simulink model "ipi_model_comparison_template"  (R2020a)
settings: Solver=ode4  StartTime=0.0  StopTime=10.0  FixedStep=1E-3  RelTol=1e-3
values from neighbouring files (symbols this model uses):
  g = 9.81    [RMIC_traj_optim_config_start.m]
  l1 = 1    [RMIC_traj_optim_config_start.m]
  lc1 = l1/2    (= 0.5)    [RMIC_traj_optim_config_start.m]
  lc2 = l2/2    (= 0.5)    [RMIC_traj_optim_config_start.m]
  m1 = 10    [RMIC_traj_optim_config_start.m]
  m2 = 10    [RMIC_traj_optim_config_start.m]
undefined symbols (not defined in the file or in its folder): beta_b, I1zz, I2zz, X
settings Model: Creator=fernando  LastModifiedBy=User
settings SFSimCC: CustomCodeUndefinedFunction=UseInterfaceOnly

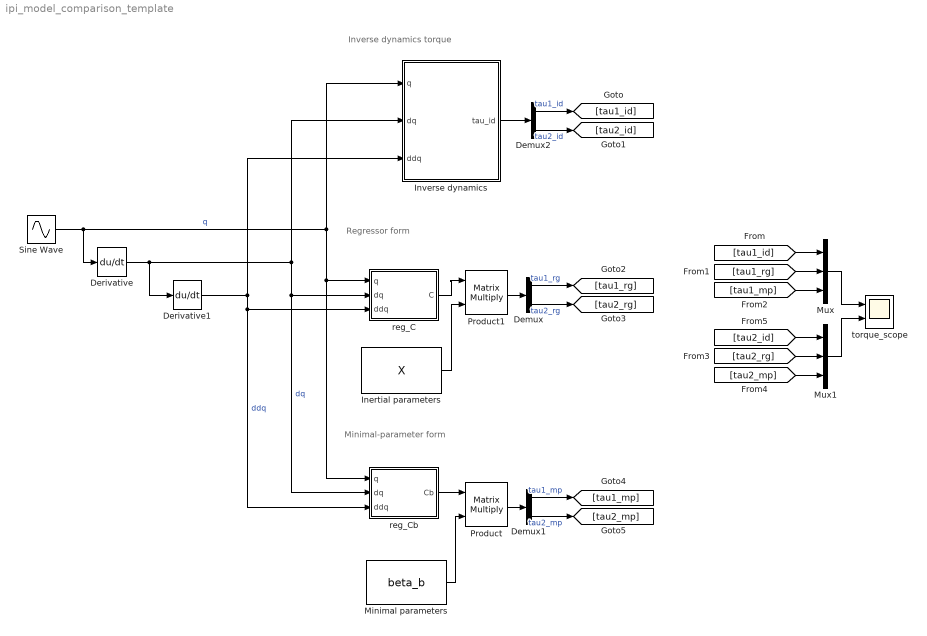
== system ipi_model_comparison_template ==
  note: Inverse dynamics torque
  note: Regressor form
  note: Minimal-parameter form
  Demux : Demux  Outputs=2
  Demux1 : Demux  Outputs=2
  Demux2 : Demux  Outputs=2
  Derivative : Derivative
  Derivative1 : Derivative
  Inertial parameters : Constant  Value=X
  Inverse dynamics : Subsystem
  Minimal parameters : Constant  Value=beta_b
  Mux : Mux  Inputs=3
  Mux1 : Mux  Inputs=3
  Product : Product  Multiplication=Matrix(*)
  Product1 : Product  Multiplication=Matrix(*)
  Sine Wave : Sin  Amplitude=[1 1]  Frequency=2*pi*(1/2)  SampleTime=0
  reg_C : MATLAB Function  TreatAsAtomicUnit=on
  reg_Cb : MATLAB Function  TreatAsAtomicUnit=on
  torque_scope : Scope  NumInputPorts=2
  wires:
  reg_Cb/1(Cb) -> Product/1
  reg_C/1(C) -> Product1/1
  Inertial parameters/1 -> Product1/2
  Sine Wave/1 -> Derivative/1, reg_Cb/1(q), reg_C/1(q), Inverse dynamics/1(q)  "q"
  Derivative/1 -> reg_Cb/2(dq), reg_C/2(dq), Inverse dynamics/2(dq), Derivative1/1  "dq"
  Derivative1/1 -> reg_Cb/3(ddq), reg_C/3(ddq), Inverse dynamics/3(ddq)  "ddq"
  Product1/1 -> Demux/1
  Product/1 -> Demux1/1
  Mux/1 -> torque_scope/1
  Mux1/1 -> torque_scope/2
  Minimal parameters/1 -> Product/2
  Demux2/1 -> [tau1_id]  "tau1_id"
  Demux2/2 -> [tau2_id]  "tau2_id"
  Demux/1 -> [tau1_rg]  "tau1_rg"
  Demux/2 -> [tau2_rg]  "tau2_rg"
  Demux1/1 -> [tau1_mp]  "tau1_mp"
  Demux1/2 -> [tau2_mp]  "tau2_mp"
  Inverse dynamics/1(tau_id) -> Demux2/1
  [tau1_id] -> Mux/1
  [tau1_rg] -> Mux/2
  [tau1_mp] -> Mux/3
  [tau2_rg] -> Mux1/2
  [tau2_mp] -> Mux1/3
  [tau2_id] -> Mux1/1

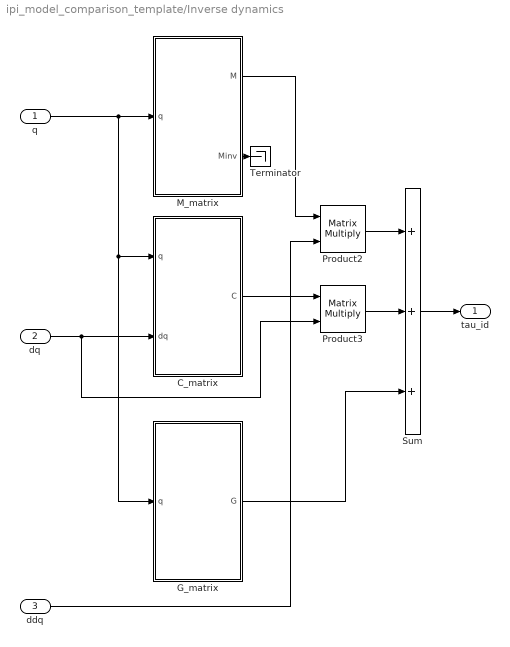
== system ipi_model_comparison_template/Inverse dynamics ==
  q : Inport
  dq : Inport  Port=2
  ddq : Inport  Port=3
  C_matrix : MATLAB Function  TreatAsAtomicUnit=on
  G_matrix : MATLAB Function  TreatAsAtomicUnit=on
  M_matrix : MATLAB Function  TreatAsAtomicUnit=on
  Product2 : Product  Multiplication=Matrix(*)
  Product3 : Product  Multiplication=Matrix(*)
  Sum : Sum  Inputs=+++
  Terminator : Terminator
  tau_id : Outport
  wires:
  M_matrix/2(Minv) -> Terminator/1
  Product2/1 -> Sum/1
  M_matrix/1(M) -> Product2/1
  dq/1 -> Product3/2, C_matrix/2(dq)
  G_matrix/1(G) -> Sum/3
  Product3/1 -> Sum/2
  q/1 -> G_matrix/1(q), C_matrix/1(q), M_matrix/1(q)
  ddq/1 -> Product2/2
  C_matrix/1(C) -> Product3/1
  Sum/1 -> tau_id/1

== matlab function ipi_model_comparison_template/reg_Cb ==
  data: q input; Cb output; dq input; ddq input
function Cb = reg_Cb(q,dq,ddq)
%#codegen

%    This function was generated by the Symbolic Math Toolbox version 8.5.
%    15-Nov-2022 11:13:43
ddq1 = ddq(1);
ddq2 = ddq(2);
dq1  = dq(1);
dq2  = dq(2);
q1   = q(1);
q2   = q(2);

t2 = cos(q2);
t3 = sin(q2);
t4 = ddq1+ddq2;
t5 = dq1+dq2;
t6 = q1+q2;
t7 = ddq1.*t2;
t8 = cos(t6);
t9 = ddq1.*t3;
t10 = sin(t6);
t11 = dq1.*dq2.*t3;
t12 = dq1.*dq2.*t2;
t13 = -t9;
t14 = -t11;
t15 = -t12;
t16 = t8.*(9.81e+2./1.0e+2);
t17 = t10.*(9.81e+2./1.0e+2);
t18 = -t17;
Cb = reshape([ddq1,0.0,cos(q1).*(9.81e+2./1.0e+2),0.0,sin(q1).*(-9.81e+2./1.0e+2),0.0,t4,t4,t7+t14+t16+t2.*t4-dq2.*t3.*t5,t7+t14+t16+dq1.*t3.*t5,t13+t15+t18-t3.*t4-dq2.*t2.*t5,t13+t15+t18+dq1.*t2.*t5],[2,6]);

== matlab function ipi_model_comparison_template/Inverse dynamics/C_matrix ==
  data: q input; C output; dq input; l1 parameter; lc2 parameter; m2 parameter
function C = C_matrix(q,dq, l1, lc2, m2)
%#codegen

%    This function was generated by the Symbolic Math Toolbox version 8.3.
%    05-Nov-2019 15:18:30

dq1  = dq(1);
dq2  = dq(2);
q1   = q(1);
q2   = q(2);

t2 = sin(q2);
C = reshape([-dq2.*l1.*lc2.*m2.*t2,dq1.*l1.*lc2.*m2.*t2,-l1.*lc2.*m2.*t2.*(dq1+dq2),0.0],[2,2]);

== matlab function ipi_model_comparison_template/Inverse dynamics/M_matrix ==
  data: M output; q input; I1zz parameter; I2zz parameter; l1 parameter; lc1 parameter; lc2 parameter; m1 parameter; m2 parameter; Minv output
function [M, Minv] = M_matrix(q, I1zz, I2zz, l1, lc1, lc2, m1, m2)
%#codegen

%    This function was generated by the Symbolic Math Toolbox version 8.3.
%    05-Nov-2019 15:18:29

q1   = q(1);
q2   = q(2);

t2 = cos(q2);
t3 = lc2.^2;
t4 = m2.*t3;
t5 = l1.*lc2.*m2.*t2;
t6 = I2zz+t4+t5;
M = reshape([I1zz+t5+t6+l1.^2.*m2+lc1.^2.*m1,t6,t6,I2zz+t4],[2,2]);
Minv = pinv(M);

== matlab function ipi_model_comparison_template/reg_C ==
  data: q input; C output; dq input; ddq input
function C = reg_C(q,dq,ddq)
%#codegen

%    This function was generated by the Symbolic Math Toolbox version 8.5.
%    15-Nov-2022 11:13:43
ddq1 = ddq(1);
ddq2 = ddq(2);
dq1  = dq(1);
dq2  = dq(2);
q1   = q(1);
q2   = q(2);

t2 = cos(q1);
t3 = cos(q2);
t4 = sin(q2);
t5 = ddq1+ddq2;
t6 = dq1+dq2;
t7 = q1+q2;
t8 = ddq1.*t3;
t9 = cos(t7);
t10 = ddq1.*t4;
t11 = sin(t7);
t12 = dq1.*dq2.*t4;
t13 = dq1.*dq2.*t3;
t17 = t2.*(9.81e+2./1.0e+2);
t14 = -t10;
t15 = -t12;
t16 = -t13;
t18 = t9.*(9.81e+2./1.0e+2);
t19 = t11.*(9.81e+2./1.0e+2);
t20 = -t19;
C = reshape([0.0,0.0,0.0,0.0,0.0,0.0,0.0,0.0,0.0,0.0,ddq1,0.0,t17,0.0,sin(q1).*(-9.81e+2./1.0e+2),0.0,0.0,0.0,0.0,0.0,0.0,0.0,0.0,0.0,0.0,0.0,0.0,0.0,0.0,0.0,t5,t5,t8+t15+t18+t3.*t5-dq2.*t4.*t6,t8+t15+t18+dq1.*t4.*t6,t14+t16+t20-t4.*t5-dq2.*t3.*t6,t14+t16+t20+dq1.*t3.*t6,0.0,0.0,ddq1+t17,0.0],[2,20]);

== matlab function ipi_model_comparison_template/Inverse dynamics/G_matrix ==
  data: G output; q input; g parameter; l1 parameter; lc1 parameter; lc2 parameter; m1 parameter; m2 parameter
function G = G_matrix(q, g, l1, lc1, lc2, m1, m2)
%#codegen

%    This function was generated by the Symbolic Math Toolbox version 8.3.
%    05-Nov-2019 15:18:30

q1   = q(1);
q2   = q(2);

t2 = cos(q1);
t3 = q1+q2;
t4 = cos(t3);
G = [g.*m2.*(l1.*t2+lc2.*t4)+g.*lc1.*m1.*t2;g.*lc2.*m2.*t4];
